simulink model "DC_motor"  (R2018a)
settings: Solver=VariableStepAuto  StartTime=0.0  StopTime=10.0  RelTol=1e-3
undefined symbols (not defined in the file): B, J, K, L, Ra
libraries: powerlib x1
settings Model: Creator=hanan  LastModifiedBy=hanan

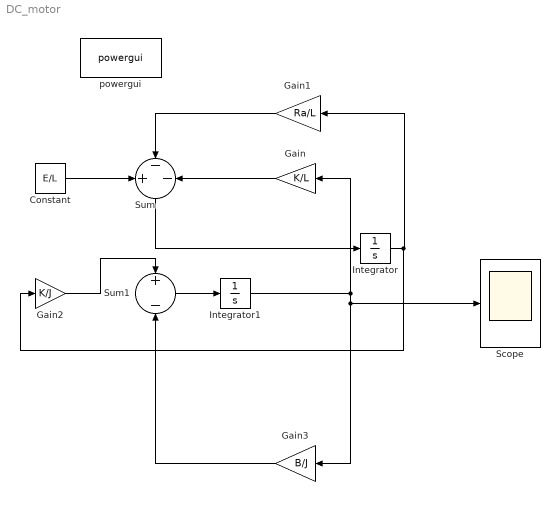
== system DC_motor ==
  Constant : Constant  Value=E/L
  Gain : Gain  Gain=K/L
  Gain1 : Gain  Gain=Ra/L
  Gain2 : Gain  Gain=K/J
  Gain3 : Gain  Gain=B/J
  Integrator : Integrator
  Integrator1 : Integrator
  Scope : Scope
  Sum : Sum  Inputs=+--
  Sum1 : Sum  Inputs=+-
  powergui : powerlib/powergui  Priority=1  SimulationMode=Continuous  SampleTime=50e-6  frequency=60  Iterations=50  frequencyindice=60  Pbase=100e6  ErrMax=1e-4  UnitsV=kV  UnitsW=MW  buscounter=0  FunctionMessages=off  echomessages=off  EnableUseOfTLC=off  CurrentSourceSwitches=off  DisableSnubberDevices=off  DisableRonSwitches=off  DisableVfSwitches=off  DisplayEquations=off  SolverType=Tustin/Backward Euler (TBE)  Interpol=off  ExternalGateDelay=off  methode=off  Ts=100  x0status=blocks  SPID=on  SwTol=0  HookPort=off  RestoreLinks=warning  ResistiveCurrentMeasurement=off  Frange=[0:2:500]  Ylog=off  Xlog=on  ShowGrid=off  save=off  variable=ZData  structure=0  ZoomFFT=off  StartTime=0.0  cycles=1  DisplayStyle=1  fundamental=60  FreqAxis=off  MaxFrequency=1000  frequencyindicesteady=1  RmsSteady=1  display=off
  wires:
  Gain/1 -> Sum/3
  Constant/1 -> Sum/1
  Gain1/1 -> Sum/2
  Integrator/1 -> Gain2/1, Gain1/1
  Gain2/1 -> Sum1/1
  Gain3/1 -> Sum1/2
  Integrator1/1 -> Scope/1, Gain3/1, Gain/1
  Sum/1 -> Integrator/1
  Sum1/1 -> Integrator1/1
